simulink model "TestLpe"  (R2020b)
settings: Solver=VariableStepAuto  StartTime=0.0  StopTime=60  RelTol=1e-3  EnableMultiTasking=on
InitFcn:
  | % load tfwt_00_run_01.mat
  | 
  | clear
  | load 2017-07-18-13-36-00_fullrate_left_right_yaw
  | if ~exist( 'logOriginal' )
  |     logOriginal = dataInOriginal
  | end
  | flog = logOriginal;
  | tSart = flog.vehicle_attitude.time(1);
  | timeStep = 0; %flog.vehicle_attitude.time(2) - flog.vehicle_attitude.time(1);
  | flog.sensor_combined.time = flog.sensor_combined.time - flog.vehicle_attitude.time(1) - timeStep;
  | flog.att_pos_mocap.time = flog.att_pos_mocap.time - flog.vehicle_attitude.time(1) - timeStep;
  | flog.control_state.time = flog.control_state.time - flog.vehicle_attitude.time(1) - timeStep;
  | flog.vehicle_local_position.time = flog.vehicle_local_position.time - flog.vehicle_attitude.time(1) - timeStep;
  | flog.vehicle_attitude.time = flog.vehicle_attitude.time - flog.vehicle_attitude.time(1);
  | 
  | tSimEnd = flog.vehicle_attitude.time(end);
(part 4 of 4)

== matlab function TestLpe/local_position_estimator/Output selection ==
  data: est_status_covariances output; est_status_health_flags output; est_status_states output; gpos_vel_n output; gpos_vel_e output; selfVec input; gpos_vel_d output; lpos_vx output; lpos_vy output; lpos_vz output; lpos_x output; lpos_y output; lpos_z output; lpos_yaw output
function [ ...
                   est_status_covariances, ...
                  est_status_health_flags, ...
                        est_status_states, ...
                               gpos_vel_n, ...
                               gpos_vel_e, ...
                               gpos_vel_d, ...
                                  lpos_vx, ...
                                  lpos_vy, ...
                                  lpos_vz, ...
                                   lpos_x, ...
                                   lpos_y, ...
                                   lpos_z, ...
                                 lpos_yaw] ...
   = OutputSelection( selfVec )
%#codegen

	% Variable assignment
	                  est_status_covariances = selfVec(439:448);
	                 est_status_health_flags = selfVec(449:449);
	                       est_status_states = selfVec(454:463);
	                              gpos_vel_n = selfVec(480:480);
	                              gpos_vel_e = selfVec(481:481);
	                              gpos_vel_d = selfVec(482:482);
	                                 lpos_vx = selfVec(501:501);
	                                 lpos_vy = selfVec(502:502);
	                                 lpos_vz = selfVec(503:503);
	                                  lpos_x = selfVec(504:504);
	                                  lpos_y = selfVec(507:507);
	                                  lpos_z = selfVec(508:508);
	                                lpos_yaw = selfVec(512:512);
end
